simulink model "Ej_pendulo"  (R2023a)
settings: Solver=VariableStepAuto  StartTime=0.0  StopTime=30  MaxStep=0.0001  RelTol=1e-3
model workspace (MAT data in the model file):
  k1 = 0.5
  m = 5
libraries: simulink x2
settings Model: Creator=santi  LastModifiedBy=santi

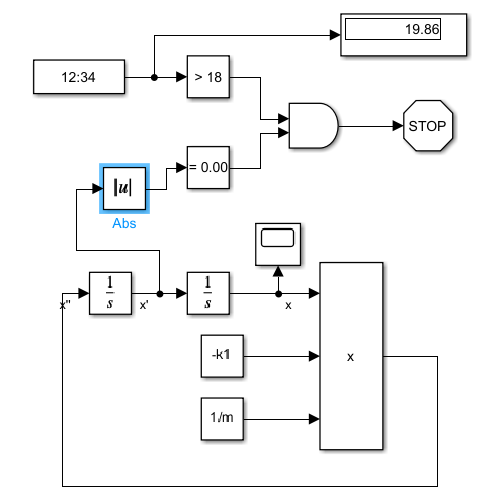
[thumbnail: Simulink's stored preview of the top-level diagram]
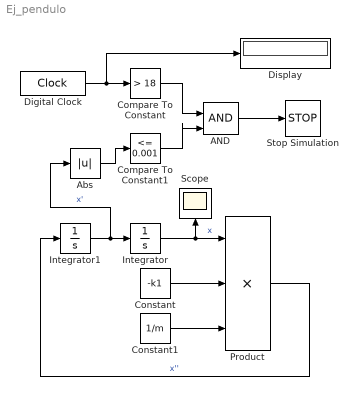
== system Ej_pendulo ==
  AND : Logic  IconShape=distinctive  AllPortsSameDT=off  OutDataTypeStr=boolean
  Abs : Abs  SaturateOnIntegerOverflow=off
  Compare To Constant : simulink/Logic and Bit Operations/Compare To Constant  relop=>  const=18  OutDataTypeStr=boolean
  Compare To Constant1 : simulink/Logic and Bit Operations/Compare To Constant  relop=<=  const=0.001  OutDataTypeStr=boolean
  Constant : Constant  Value=-k1
  Constant1 : Constant  Value=1/m
  Digital Clock : DigitalClock  SampleTime=0.001
  Display : Display
  Integrator : Integrator  InitialCondition=1.5
  Integrator1 : Integrator
  Product : Product  Inputs=3
  Scope : Scope
  Stop Simulation : Stop
  wires:
  Integrator1/1 -> Abs/1, Integrator/1  "x'"
  Integrator/1 -> Product/1, Scope/1  "x"
  Product/1 -> Integrator1/1  "x''"
  Constant/1 -> Product/2
  Constant1/1 -> Product/3
  Digital Clock/1 -> Display/1, Compare To Constant/1
  Compare To Constant/1 -> AND/1
  Compare To Constant1/1 -> AND/2
  AND/1 -> Stop Simulation/1
  Abs/1 -> Compare To Constant1/1
